simulink model "ej2"  (R2019a)
settings: Solver=ode3  StartTime=0.0  StopTime=100.0  FixedStep=0.01  RelTol=1e-3
undefined symbols (not defined in the file or in its folder): DiscIntNeverNeededParam
libraries: simulink x1
settings Model: EnablePacing=on  Creator=tromp  LastModifiedBy=tromp
settings DataIOCC: ReturnWorkspaceOutputs=off

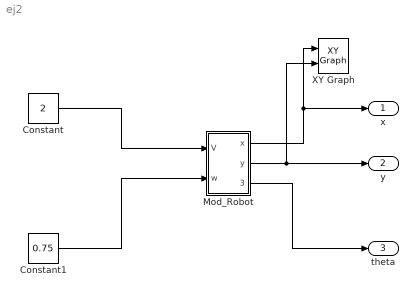
== system ej2 ==
  Constant : Constant  Value=2
  Constant1 : Constant  Value=0.75
  Mod_Robot : Subsystem
  XY Graph : simulink/Sinks/XY Graph  xmin=-10  xmax=10  ymin=-10  ymax=10  st=0.01
  x : Outport
  y : Outport  Port=2
  "theta " : Outport  Port=3
  wires:
  Constant/1 -> Mod_Robot/1(V)
  Constant1/1 -> Mod_Robot/2(w)
  Mod_Robot/1(x) -> XY Graph/1, x/1
  Mod_Robot/2(y) -> XY Graph/2, y/1
  Mod_Robot/3("theta ") -> "theta "/1

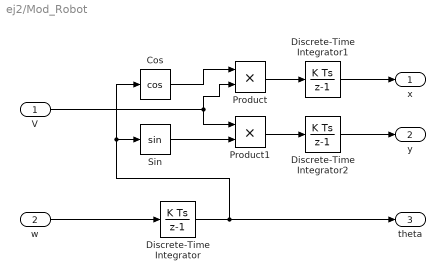
== system ej2/Mod_Robot ==
  V : Inport
  w : Inport  Port=2
  Cos : Trigonometry  Operator=cos
  Discrete-Time Integrator : DiscreteIntegrator  InitialCondition=30*pi/180  SampleTime=0.01  ICPrevOutput=DiscIntNeverNeededParam  ICPrevScaledInput=DiscIntNeverNeededParam
  Discrete-Time Integrator1 : DiscreteIntegrator  InitialCondition=-4  SampleTime=0.01  ICPrevOutput=DiscIntNeverNeededParam  ICPrevScaledInput=DiscIntNeverNeededParam
  Discrete-Time Integrator2 : DiscreteIntegrator  InitialCondition=-4  SampleTime=0.01  ICPrevOutput=DiscIntNeverNeededParam  ICPrevScaledInput=DiscIntNeverNeededParam
  Product : Product
  Product1 : Product
  Sin : Trigonometry
  x : Outport
  y : Outport  Port=2
  "theta " : Outport  Port=3
  wires:
  Discrete-Time Integrator/1 -> "theta "/1, Cos/1, Sin/1
  Cos/1 -> Product/1
  Product1/1 -> Discrete-Time Integrator2/1
  Product/1 -> Discrete-Time Integrator1/1
  Discrete-Time Integrator1/1 -> x/1
  V/1 -> Product/2, Product1/1
  Discrete-Time Integrator2/1 -> y/1
  Sin/1 -> Product1/2
  w/1 -> Discrete-Time Integrator/1
